simulink model "simple_pendulum"  (R2017b)
settings: Solver=FixedStepAuto  StartTime=0.0  StopTime=30  FixedStep=0.1  RelTol=1e-3
undefined symbols (not defined in the file or in its folder): B, g, l, m
settings Model: Creator=ArsalanBangash  LastModifiedBy=ArsalanBangash

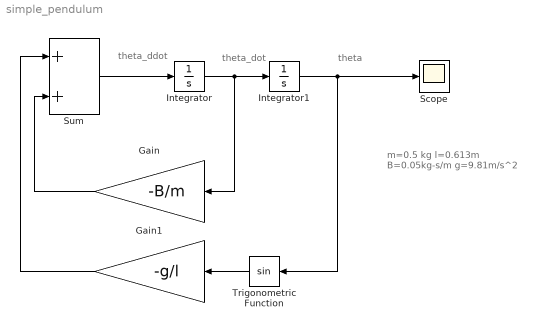
== system simple_pendulum ==
  note: m=0.5 kg
      | l=0.613m
      | B=0.05kg-s/m
      | g=9.81m/s^2
  note: theta
  note: theta_dot
  note: theta_ddot
  Gain : Gain  Gain=-B/m
  Gain1 : Gain  Gain=-g/l
  Integrator : Integrator  InitialCondition=1
  Integrator1 : Integrator
  Scope : Scope
  Sum : Sum  Inputs=|++
  Trigonometric Function : Trigonometry
  wires:
  Sum/1 -> Integrator/1
  Integrator/1 -> Gain/1, Integrator1/1
  Integrator1/1 -> Trigonometric Function/1, Scope/1
  Gain/1 -> Sum/2
  Gain1/1 -> Sum/1
  Trigonometric Function/1 -> Gain1/1
